simulink library "linera_full_oredr_observer"  (R2021a)
settings: Solver=VariableStepAuto  StartTime=0.0  StopTime=10.0  RelTol=1e-3
values from neighbouring files (symbols this model uses):
  A = [0    1     0    0 ... (first row only)    [state_space_matrices.m]
  B = [0 0;1/m1 0;0 0;0 1/m2]    [state_space_matrices.m]
  C_1 = eye(4)    [state_space_matrices.m]
  D_1 = zeros(4, 2)    [state_space_matrices.m]
  Kf_1 = lqr(A',C_1',Q,R)'    [state_space_matrices.m]
settings Model: Creator=husse  LastModifiedBy=husse

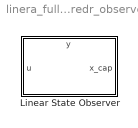
== system linera_full_oredr_observer ==
  Linear State Observer : Subsystem  mask{A_marix=A, B_matrix=B, C_matrix=C_1, D_matrix=D_1, K_matrix=Kf_1, IC=0}
      mask prompts: A_marix "A"; B_matrix "B"; C_matrix "C"; D_matrix "D"; K_matrix "K"; IC "initial condition"
      settings: PortSchema="{\"entries\":[{\"content\":{\"sides\":[{\"content\":{\"connectorIds\":[\"In1\"]},\"type\":\"ConnectorPlacement.EquallySpacedRectSide\",\"uuid\":\"986d422d-b8ff-4d9a-baf2-00a8ac9f9019\"},{\"content\":{\"connectorIds\":[\"Out1\"],\"side\":\"RIGHT\"},\"type\":\"ConnectorPlacement.EquallySpacedRectSide\",\"uuid\":\"59e96993-3a48-4151-9be3-a9dc09e1e33d\"},{\"content\":{\"connectorIds\":[\"In2\"],\"side\":\"TOP\"},\"type\":\"ConnectorPlacement.EquallySpacedRectSide\",\"uuid\":\"13ba996f-1b17-4586-8eaf-63e69bc07399\"}]},\"type\":\"ConnectorPlacement.EquallySpacedConnector\",\"uuid\":\"b109a439-7035-48cd-b1f6-10e4a3832946\"}],\"packageUris\":[\"http://schema.mathworks.com/mf0/Connector/R2020b\"],\"version\":\"1.0\"}"

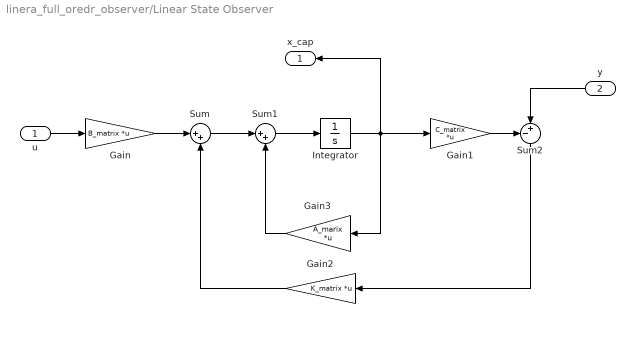
== system linera_full_oredr_observer/Linear State Observer ==
  u : Inport
  y : Inport  Port=2
  Gain : Gain  Gain=B_matrix  Multiplication=Matrix(K*u)
  Gain1 : Gain  Gain=C_matrix  Multiplication=Matrix(K*u)
  Gain2 : Gain  Gain=K_matrix  Multiplication=Matrix(K*u)
  Gain3 : Gain  Gain=A_marix  Multiplication=Matrix(K*u)
  Integrator : Integrator  InitialCondition=IC
  Sum : Sum  Inputs=|++
  Sum1 : Sum  Inputs=|++
  Sum2 : Sum  Inputs=-+|
  x_cap : Outport
  wires:
  Gain2/1 -> Sum/2
  Sum2/1 -> Gain2/1
  Gain1/1 -> Sum2/1
  Integrator/1 -> x_cap/1, Gain3/1, Gain1/1
  Sum/1 -> Sum1/1
  Sum1/1 -> Integrator/1
  Gain3/1 -> Sum1/2
  Gain/1 -> Sum/1
  y/1 -> Sum2/2
  u/1 -> Gain/1
